simulink model "FlightGear_BUS_aerosurface_trim"  (R2017a)
settings: Solver=VariableStepAuto  StartTime=0.0  StopTime=20  FixedStep=0.1  RelTol=1e-5
model workspace (MAT data in the model file):
  op_trim2 : opcond.OperatingReport (value not decoded)
  op_trim3 : opcond.OperatingReport (value not decoded)
values from neighbouring files (symbols this model uses):
  a0_s2345 = [0;0;0.05;0.05]    [HW5_4_surfaces.m]    (also in TEST_aerosetup.m; surfaces_setup_test.m)
  A_2345 = c_2345.*b_2345    [HW5_4_surfaces.m]    (also in TEST_aerosetup.m; surfaces_setup_test.m)
  Aileron_left = 0    [HW5_4_surfaces.m]    (also in TEST_aerosetup.m; surfaces_setup_test.m)
  Aileron_right = 0    [HW5_4_surfaces.m]    (also in TEST_aerosetup.m; surfaces_setup_test.m)
  c_2345 = [0.075;0.08;0.1;0.1]    [HW5_4_surfaces.m]    (also in TEST_aerosetup.m; surfaces_setup_test.m)
  CD0_s2345 = [0.01;0.01;0.01;0.01]    [HW5_4_surfaces.m]    (also in TEST_aerosetup.m; surfaces_setup_test.m)
  CDa_s2345 = [1;1;1;1]    [HW5_4_surfaces.m]    (also in TEST_aerosetup.m; surfaces_setup_test.m)
  CL0_2345 = [0;0; 0.05; 0.05]    [HW5_4_surfaces.m]    (also in TEST_aerosetup.m; surfaces_setup_test.m)
  CLa = 2*pi*(r./(2+r))    [HW5_4_surfaces.m]    (also in TEST_aerosetup.m; surfaces_setup_test.m)
  CM0_s2345 = [0;0;-0.05;-0.05]    [HW5_4_surfaces.m]    (also in TEST_aerosetup.m; surfaces_setup_test.m)
  CMa_s2345 = [0; 0; 0; 0]    [HW5_4_surfaces.m]    (also in TEST_aerosetup.m; surfaces_setup_test.m)
  e_s2345 = [0.8;0.8;0.9;0.9]    [HW5_4_surfaces.m]    (also in TEST_aerosetup.m; surfaces_setup_test.m)
  elevator = 0    [HW5_4_surfaces.m]    (also in TEST_aerosetup.m; surfaces_setup_test.m)
  Fext_N = -g_EN * m    [HW5_4_surfaces.m]    (also in TEST_aerosetup.m = [10 10 10]; surfaces_setup_test.m)
  g_EN = [0; 0; 9.81]    [HW5_4_surfaces.m]    (also in TEST_aerosetup.m = [0; 0; 9.8]; surfaces_setup_test.m)
  i_s2345 = [0; 0; 0.05; 0.05;]    [HW5_4_surfaces.m]    (also in TEST_aerosetup.m; surfaces_setup_test.m)
  J_cg = ones(3)    [HW5_4_surfaces.m]    (also in TEST_aerosetup.m)
  J_cgp = ones(3)    [surfaces_setup_test.m]
  M_total = sum(MnG(:,1))/1000    [HW5_4_surfaces.m]    (also in TEST_aerosetup.m; surfaces_setup_test.m = sum(MnG1(:,1))/1000)
  Mext_B = [0; 0; 0]    [HW5_4_surfaces.m]    (also in TEST_aerosetup.m = [1; 1; 1]; surfaces_setup_test.m)
  p_E_BE_ini = p_E_BE_ini_deg .* [deg2rad; deg2rad; 1]    [HW5_4_surfaces.m]    (also in TEST_aerosetup.m; surfaces_setup_test.m)
  r = b_2345./c_2345    [HW5_4_surfaces.m]    (also in TEST_aerosetup.m; surfaces_setup_test.m)
  Rearth = 6371000    [HW5_4_surfaces.m]    (also in TEST_aerosetup.m; surfaces_setup_test.m)
  rudder = 0    [HW5_4_surfaces.m]    (also in TEST_aerosetup.m; surfaces_setup_test.m)
  Theta_ini = Theta_ini_deg * deg2rad    [HW5_4_surfaces.m]    (also in TEST_aerosetup.m; surfaces_setup_test.m)
  v_N_AE = [0;0;0]    [HW5_4_surfaces.m]    (also in TEST_aerosetup.m; surfaces_setup_test.m)
  Vbbe_int = [10; 0; 0]    [HW5_4_surfaces.m]    (also in TEST_aerosetup.m; surfaces_setup_test.m = [5; 0; 0])
  w_B_BE_ini = [1e0; 1e-2; 1e-2]    [HW5_4_surfaces.m]    (also in TEST_aerosetup.m; surfaces_setup_test.m)
  xyz_s = [[-0.76 0 0.16];[-0.76 0 -0.09];[-0.23 0.44 0];[-0.23 -0.44 0];]    [HW5_4_surfaces.m]    (also in TEST_aerosetup.m; surfaces_setup_test.m)
undefined symbols (not defined in the file or in its folder): Earth, WGS84
libraries: dspinverses x6, vrlib x4, simulink x4, aerolibfltsims x3, sharedtransform x2, aerolibtransform2 x2, aerolibutil x1, sharedutil x1
(part 1 of 2)
settings Model: Creator=Jiaoran Wang  LastModifiedBy=Jiaoran Wang
settings DataIOCC: ExternalInput=getinputstruct(op_trim3)  InitialState=getstatestruct(op_trim3)  LoadExternalInput=on  LoadInitialState=on

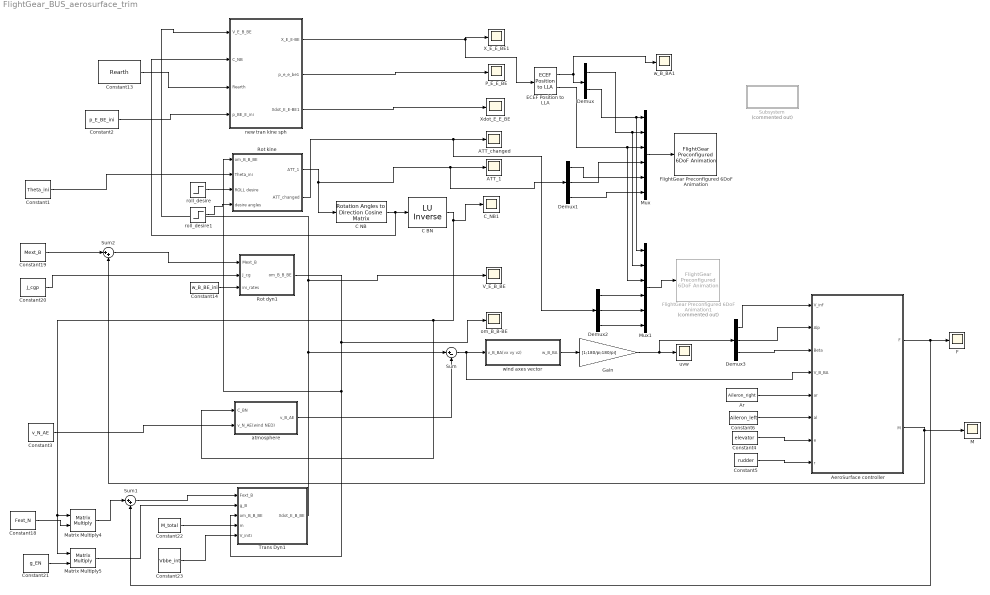
== system FlightGear_BUS_aerosurface_trim ==
  ATT_1 : Scope
  ATT_changed : Scope
  AeroSurface controller : Subsystem
  Ar : Constant  Value=Aileron_right
  C BN : dspinverses/ LU Inverse
      settings: SourceProductName=DSP System Toolbox
  C NB : sharedtransform/Rotation Angles to Direction Cosine Matrix  rotationOrder=ZYX
  C_NB1 : Scope
  Constant1 : Constant  Value=Theta_ini
  Constant13 : Constant  Value=Rearth
  Constant14 : Constant  Value=w_B_BE_ini
  Constant18 : Constant  Value=Fext_N
  Constant19 : Constant  Value=Mext_B
  Constant2 : Constant  Value=p_E_BE_ini  VectorParams1D=off
  Constant20 : Constant  Value=J_cgp
  Constant21 : Constant  Value=g_EN
  Constant22 : Constant  Value=M_total
  Constant23 : Constant  Value=Vbbe_int
  Constant3 : Constant  Value=v_N_AE
  Constant4 : Constant  Value=elevator
  Constant5 : Constant  Value=rudder
  Constant6 : Constant  Value=Aileron_left
  Demux : Demux  Outputs=2
  Demux1 : Demux  Outputs=3
  Demux2 : Demux  Outputs=3
  Demux3 : Demux  Outputs=3
  ECEF Position to LLA : aerolibtransform2/ECEF Position to LLA  units=Metric (MKS)  ptype=Earth (WGS84)  F=1/298.257223563  R=6378137
      settings: SourceProductName=Aerospace Blockset  SourceProductBaseCode=AE
  F : Scope
  FlightGear Preconfigured 6DoF Animation : aerolibfltsims/FlightGear Preconfigured 6DoF Animation  xFlightGearVersion=v3.0  DestinationIpAddress=127.0.0.1  DestinationPort=5502  SampleTime=1/50
      settings: SourceProductName=Aerospace Blockset
  FlightGear Preconfigured 6DoF Animation1 : aerolibfltsims/FlightGear Preconfigured 6DoF Animation  Commented=on  xFlightGearVersion=v3.0  DestinationIpAddress=127.0.0.1  DestinationPort=5502  SampleTime=1/50
      settings: SourceProductName=Aerospace Blockset
  Gain : Gain  Gain=[1;180/pi;180/pi]
  M : Scope
  Matrix Multiply4 : Product  Multiplication=Matrix(*)
  Matrix Multiply5 : Product  Multiplication=Matrix(*)
  Mux : Mux  Inputs=6
  Mux1 : Mux  Inputs=6
  P_E_E_BE : Scope
  Rot dyn1 : Subsystem
  Rot kine : Subsystem
  Subsystem : Subsystem  Commented=on
  Sum : Sum  Inputs=|+-
  Sum1 : Sum  Inputs=|++
  Sum2 : Sum  Inputs=|++
  Trans Dyn1 : Subsystem
  V_E_B_BE : Scope
  "X_E_E_BE1 " : Scope
  Xdot_E_E_BE : Scope
  atmosphere : Subsystem
  new tran kine sph : Subsystem
  om_B_B-BE : Scope
  roll_desire : Step  Time=0  After=0  SampleTime=0
  roll_desire1 : Step  Time=0  After=0  SampleTime=0
  uvw : Scope
  w_B_BA1 : Scope
  wind axes vector : Subsystem
  wires:
  ECEF Position to LLA/1 -> Demux/1, w_B_BA1/1
  Constant2/1 -> new tran kine sph/4(p_BE_E_ini)
  Constant13/1 -> new tran kine sph/3(Rearth)
  C BN/1 -> C_NB1/1, atmosphere/1(C_BN), Matrix Multiply5/1, Matrix Multiply4/1
  Matrix Multiply5/1 -> Trans Dyn1/2(g_B)
  Demux/1 -> Mux1/2, Mux/2
  new tran kine sph/2(p_e_e_be1) -> P_E_E_BE/1
  Constant23/1 -> Trans Dyn1/5(V_initi)
  ECEF Position to LLA/2 -> Mux1/3, Mux/3
  Constant18/1 -> Matrix Multiply4/2
  wind axes vector/1(w_B_BA) -> Gain/1
  atmosphere/1(v_B_AE) -> Sum/2
  Demux/2 -> Mux1/1, Mux/1
  Constant3/1 -> atmosphere/2(v_N_AE(wind NED))
  new tran kine sph/1(X_E_E-BE) -> "X_E_E_BE1 "/1, ECEF Position to LLA/1
  new tran kine sph/3(Xdot_E_E-BE1) -> Xdot_E_E_BE/1
  Rot dyn1/1(om_B_B_BE) -> Trans Dyn1/3(om_B_B_BE), Rot kine/1(om_B_B_BE), om_B_B-BE/1
  Constant14/1 -> Rot dyn1/3(ini_rates)
  Constant1/1 -> Rot kine/2(Theta_ini)
  Trans Dyn1/1(Xdot_E_B_BE) -> new tran kine sph/1(V_E_B_BE), V_E_B_BE/1, Sum/1
  Constant22/1 -> Trans Dyn1/4(m)
  Constant21/1 -> Matrix Multiply5/2
  C NB/1 -> new tran kine sph/2(C_NB), C BN/1
  Rot kine/1(ATT_1) -> Demux1/1, ATT_1/1, C NB/1
  Constant20/1 -> Rot dyn1/2(J_cg)
  Mux/1 -> FlightGear Preconfigured 6DoF Animation/1
  Demux1/3 -> Mux/6
  Rot kine/2(ATT_changed) -> Demux2/1, ATT_changed/1
  roll_desire/1 -> Rot kine/3(ROLL desire)
  roll_desire1/1 -> Rot kine/4(" desire angles")
  Mux1/1 -> FlightGear Preconfigured 6DoF Animation1/1
  Demux2/3 -> Mux1/6
  Demux2/2 -> Mux1/5
  Demux2/1 -> Mux1/4
  Demux1/2 -> Mux/4
  Demux1/1 -> Mux/5
  Gain/1 -> Demux3/1, uvw/1
  Demux3/1 -> AeroSurface controller/1(V_inf)
  Demux3/2 -> AeroSurface controller/2(Alp)
  Demux3/3 -> AeroSurface controller/3(Beta)
  Sum/1 -> AeroSurface controller/4(V_B_BA), wind axes vector/1(v_B_BA(vx vy vz))
  Constant4/1 -> AeroSurface controller/7(e)
  Constant5/1 -> AeroSurface controller/8(r)
  Ar/1 -> AeroSurface controller/5(ar)
  Constant6/1 -> AeroSurface controller/6(al)
  AeroSurface controller/2(M) -> M/1, Sum2/2
  Matrix Multiply4/1 -> Sum1/1
  Sum1/1 -> Trans Dyn1/1(Fext_B)
  AeroSurface controller/1(F) -> F/1, Sum1/2
  Constant19/1 -> Sum2/1
  Sum2/1 -> Rot dyn1/1(Mext_B)

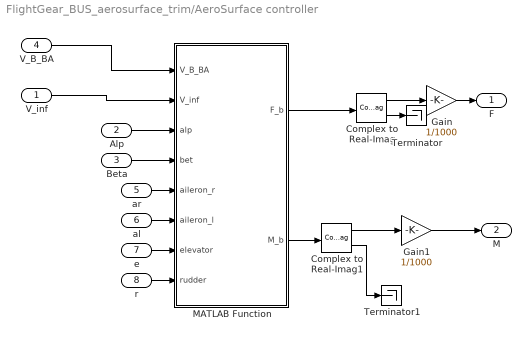
== system FlightGear_BUS_aerosurface_trim/AeroSurface controller ==
  V_inf : Inport
  Alp : Inport  Port=2
  Beta : Inport  Port=3
  V_B_BA : Inport  Port=4
  ar : Inport  Port=5
  al : Inport  Port=6
  e : Inport  Port=7
  r : Inport  Port=8
  Complex to Real-Imag : ComplexToRealImag
  Complex to Real-Imag1 : ComplexToRealImag
  Gain : Gain  Gain=1/1000
  Gain1 : Gain  Gain=1/1000
  MATLAB Function : MATLAB Function  TreatAsAtomicUnit=on
  Terminator : Terminator
  Terminator1 : Terminator
  F : Outport
  M : Outport  Port=2
  wires:
  V_inf/1 -> MATLAB Function/2(V_inf)
  V_B_BA/1 -> MATLAB Function/1(V_B_BA)
  ar/1 -> MATLAB Function/5(aileron_r)
  al/1 -> MATLAB Function/6(aileron_l)
  e/1 -> MATLAB Function/7(elevator)
  r/1 -> MATLAB Function/8(rudder)
  Alp/1 -> MATLAB Function/3(alp)
  Beta/1 -> MATLAB Function/4(bet)
  MATLAB Function/1(F_b) -> Complex to Real-Imag/1
  Complex to Real-Imag/1 -> Gain/1
  Complex to Real-Imag/2 -> Terminator/1
  MATLAB Function/2(M_b) -> Complex to Real-Imag1/1
  Complex to Real-Imag1/2 -> Terminator1/1
  Complex to Real-Imag1/1 -> Gain1/1
  Gain/1 -> F/1
  Gain1/1 -> M/1

== system FlightGear_BUS_aerosurface_trim/Rot dyn1 ==
  Mext_B : Inport
  J_cg : Inport  Port=2
  ini_rates : Inport  Port=3
  " LU Inverse" : dspinverses/ LU Inverse
      settings: SourceProductName=DSP System Toolbox
  Add : Sum  Inputs=+-
  Cross Product : vrlib/Utilities/Cross Product
      settings: SourceProductBaseCode=VR
  Integrator : Integrator  InitialConditionSource=external
  Matrix Multiply : Product  Multiplication=Matrix(*)
  Matrix Multiply1 : Product  Multiplication=Matrix(*)
  om_B_B_BE : Outport
  wires:
  J_cg/1 -> " LU Inverse"/1, Matrix Multiply/1
  Matrix Multiply/1 -> Cross Product/2
  " LU Inverse"/1 -> Matrix Multiply1/1
  Add/1 -> Matrix Multiply1/2
  Cross Product/1 -> Add/2
  Matrix Multiply1/1 -> Integrator/1
  ini_rates/1 -> Integrator/2
  Integrator/1 -> Cross Product/1, Matrix Multiply/2, om_B_B_BE/1
  Mext_B/1 -> Add/1

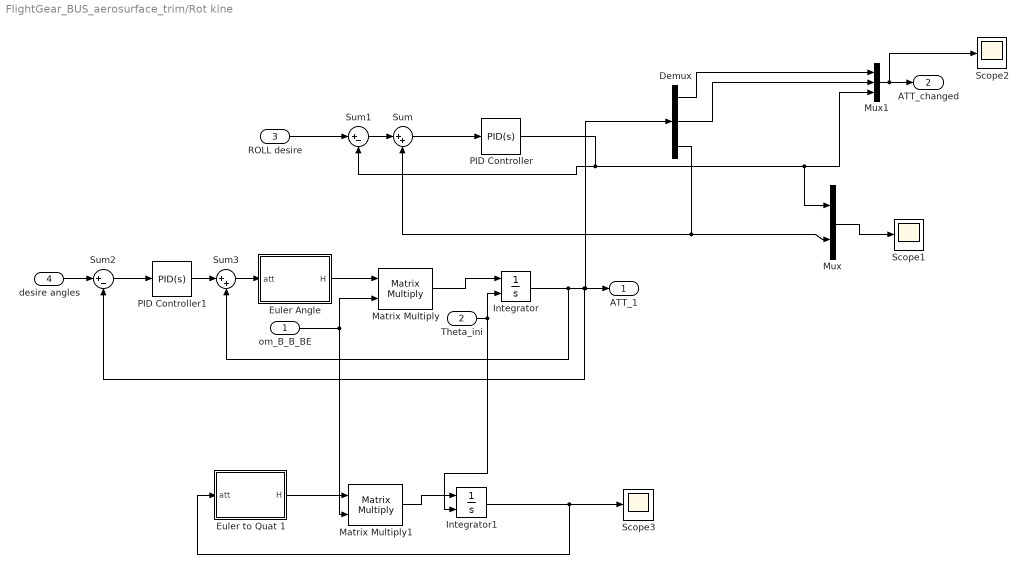
== system FlightGear_BUS_aerosurface_trim/Rot kine ==
  om_B_B_BE : Inport
  Theta_ini : Inport  Port=2
  ROLL desire : Inport  Port=3
  " desire angles" : Inport  Port=4
  Demux : Demux  Outputs=3
  "Euler Angle " : MATLAB Function  TreatAsAtomicUnit=on
  Euler to Quat 1 : MATLAB Function  TreatAsAtomicUnit=on
  Integrator : Integrator  InitialConditionSource=external
  Integrator1 : Integrator  InitialConditionSource=external
  Matrix Multiply : Product  Multiplication=Matrix(*)
  Matrix Multiply1 : Product  Multiplication=Matrix(*)
  Mux : Mux  Inputs=2
  Mux1 : Mux  Inputs=3
  PID Controller : simulink/Continuous/PID Controller  Controller=PID  TimeDomain=Continuous-time  SampleTime=-1  IntegratorMethod=Forward Euler  FilterMethod=Forward Euler  Form=Parallel  UseFilter=on  ControllerParametersSource=internal  P=0  I=10  D=0  N=100  InitialConditionSource=internal  InitialConditionForIntegrator=0  InitialConditionForFilter=0  ExternalReset=none  LimitOutput=off  UpperSaturationLimit=inf  LowerSaturationLimit=-inf  LinearizeAsGain=on  AntiWindupMode=none  Kb=1  TrackingMode=off  Kt=1  PParamMin=[]  PParamMax=[]  IParamMin=[]  IParamMax=[]  DParamMin=[]  DParamMax=[]  NParamMin=[]  NParamMax=[]  KbParamMin=[]  KbParamMax=[]  KtParamMin=[]  KtParamMax=[]  POutMin=[]  POutMax=[]  IOutMin=[]  IOutMax=[]  DOutMin=[]  DOutMax=[]  NOutMin=[]  NOutMax=[]  KbOutMin=[]  KbOutMax=[]  KtOutMin=[]  KtOutMax=[]  IntegratorOutMin=[]  IntegratorOutMax=[]  FilterOutMin=[]  FilterOutMax=[]  SumOutMin=[]  SumOutMax=[]  SumI1OutMin=[]  SumI1OutMax=[]  SumI2OutMin=[]  SumI2OutMax=[]  SumI3OutMin=[]  SumI3OutMax=[]  SumDOutMin=[]  SumDOutMax=[]  SaturationOutMin=[]  SaturationOutMax=[]  IntegratorContinuousStateAttributes=''  IntegratorStateMustResolveToSignalObject=off  IntegratorRTWStateStorageClass=Auto  FilterContinuousStateAttributes=''  FilterStateMustResolveToSignalObject=off  FilterRTWStateStorageClass=Auto  DifferentiatorICPrevScaledInput=0  DifferentiatorOutMin=[]  DifferentiatorOutMax=[]  InitialConditionSetting=State (most efficient)
  PID Controller1 : simulink/Continuous/PID Controller  Controller=PID  TimeDomain=Continuous-time  SampleTime=-1  IntegratorMethod=Forward Euler  FilterMethod=Forward Euler  Form=Parallel  UseFilter=on  ControllerParametersSource=internal  P=0  I=10  D=0  N=100  InitialConditionSource=internal  InitialConditionForIntegrator=0  InitialConditionForFilter=0  ExternalReset=none  LimitOutput=off  UpperSaturationLimit=inf  LowerSaturationLimit=-inf  LinearizeAsGain=on  AntiWindupMode=none  Kb=1  TrackingMode=off  Kt=1  PParamMin=[]  PParamMax=[]  IParamMin=[]  IParamMax=[]  DParamMin=[]  DParamMax=[]  NParamMin=[]  NParamMax=[]  KbParamMin=[]  KbParamMax=[]  KtParamMin=[]  KtParamMax=[]  POutMin=[]  POutMax=[]  IOutMin=[]  IOutMax=[]  DOutMin=[]  DOutMax=[]  NOutMin=[]  NOutMax=[]  KbOutMin=[]  KbOutMax=[]  KtOutMin=[]  KtOutMax=[]  IntegratorOutMin=[]  IntegratorOutMax=[]  FilterOutMin=[]  FilterOutMax=[]  SumOutMin=[]  SumOutMax=[]  SumI1OutMin=[]  SumI1OutMax=[]  SumI2OutMin=[]  SumI2OutMax=[]  SumI3OutMin=[]  SumI3OutMax=[]  SumDOutMin=[]  SumDOutMax=[]  SaturationOutMin=[]  SaturationOutMax=[]  IntegratorContinuousStateAttributes=''  IntegratorStateMustResolveToSignalObject=off  IntegratorRTWStateStorageClass=Auto  FilterContinuousStateAttributes=''  FilterStateMustResolveToSignalObject=off  FilterRTWStateStorageClass=Auto  DifferentiatorICPrevScaledInput=0  DifferentiatorOutMin=[]  DifferentiatorOutMax=[]  InitialConditionSetting=State (most efficient)
  Scope1 : Scope
  Scope2 : Scope
  Scope3 : Scope
  Sum : Sum  Inputs=|++
  Sum1 : Sum  Inputs=|+-
  Sum2 : Sum  Inputs=|+-
  Sum3 : Sum  Inputs=|++
  ATT_1 : Outport
  ATT_changed : Outport  Port=2
  wires:
  om_B_B_BE/1 -> Matrix Multiply1/2, Matrix Multiply/2
  Integrator/1 -> ATT_1/1, Demux/1, Sum2/2, Sum3/2
  "Euler Angle "/1(H) -> Matrix Multiply/1
  Theta_ini/1 -> Integrator/2, Integrator1/2
  Matrix Multiply/1 -> Integrator/1
  Demux/3 -> Sum/2, Mux/2
  Demux/1 -> Mux1/1
  PID Controller/1 -> Sum1/2, Mux/1, Mux1/3
  Mux/1 -> Scope1/1
  Demux/2 -> Mux1/2
  Mux1/1 -> Scope2/1, ATT_changed/1
  ROLL desire/1 -> Sum1/1
  Sum1/1 -> Sum/1
  Sum/1 -> PID Controller/1
  Sum2/1 -> PID Controller1/1
  " desire angles"/1 -> Sum2/1
  PID Controller1/1 -> Sum3/1
  Sum3/1 -> "Euler Angle "/1(att)
  Integrator1/1 -> Euler to Quat 1/1(att), Scope3/1
  Matrix Multiply1/1 -> Integrator1/1
  Euler to Quat 1/1(H) -> Matrix Multiply1/1

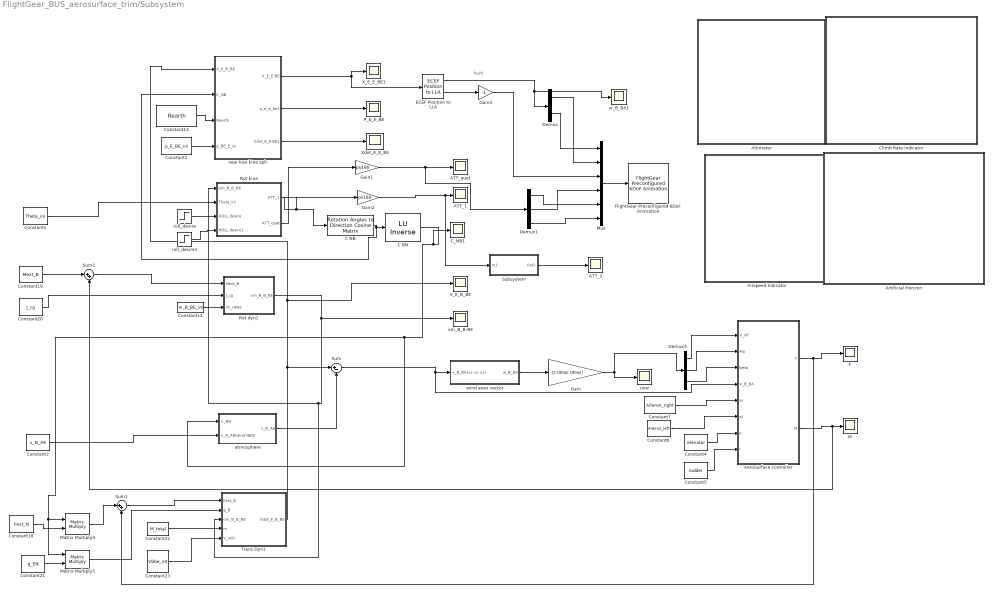
== system FlightGear_BUS_aerosurface_trim/Subsystem ==
  note: hurh
  ATT_1 : Scope
  ATT_2 : Scope
  ATT_quat : Scope
  AeroSurface controller : Subsystem
  Airspeed Indicator : Subsystem  DialogController=aeroblksHMICreateDDGDialog  IsWebBlock=on  mask(MWDashboardBlock){webBlockId=e5e3171d-ff29-4451-bf74-d38876eec561, webBlockType=airspeedindicator, ShowInLibBrowser=on, ShowInitialText=on, HMISrcModelName=[]}
      mask prompts: webBlockId "WebBlock Id"; webBlockType "WebBlock Type"; HMISrcModelName "Source Model"
      mask help: aeroblksHMI:aeroblkhmi:AirspeedIndicatorDialogDesc
      mask Help: eval('asbhmihelp(''airspeedindicator'')');
      mask Display:
      | if strcmp(get_param(bdroot(gcb),'BlockDiagramType'), 'library')
      |  image([(matlabroot) '/toolbox/aeroblks/aeroblks/hmi/icons/AirspeedIndicatorIcon.svg'])
      | end
  Altimeter : Subsystem  DialogController=aeroblksHMICreateDDGDialog  IsWebBlock=on  mask(MWDashboardBlock){webBlockId=36990637-e96a-433a-956a-f44ed4ed9d1e, webBlockType=altimeter, ShowInLibBrowser=on, ShowInitialText=on, HMISrcModelName=[]}
      mask prompts: webBlockId "WebBlock Id"; webBlockType "WebBlock Type"; HMISrcModelName "Source Model"
      mask help: aeroblksHMI:aeroblkhmi:AltimeterDialogDesc
      mask Help: eval('asbhmihelp(''altimeter'')');
      mask Display:
      | if strcmp(get_param(bdroot(gcb),'BlockDiagramType'), 'library')
      |  image([(matlabroot) '/toolbox/aeroblks/aeroblks/hmi/icons/AltimeterIcon.svg'])
      | end
  Artificial Horizon : Subsystem  DialogController=aeroblksHMICreateDDGDialog  IsWebBlock=on  mask(MWDashboardBlock){webBlockId=4cd5d09c-38f7-433d-892c-50154f5485b8, webBlockType=artificialhorizon, ShowInLibBrowser=on, ShowInitialText=on, HMISrcModelName=[]}
      mask prompts: webBlockId "WebBlock Id"; webBlockType "WebBlock Type"; HMISrcModelName "Source Model"
      mask help: aeroblksHMI:aeroblkhmi:ArtificialHorizonDialogDesc
      mask Help: eval('asbhmihelp(''artificialhorizon'')');
      mask Display:
      | if strcmp(get_param(bdroot(gcb),'BlockDiagramType'), 'library')
      |  image([(matlabroot) '/toolbox/aeroblks/aeroblks/hmi/icons/ArtificialHorizonIcon.svg'])
      | end
  C BN : dspinverses/ LU Inverse
      settings: SourceProductName=DSP System Toolbox
  C NB : sharedtransform/Rotation Angles to Direction Cosine Matrix  rotationOrder=ZYX
  C_NB1 : Scope
  Climb Rate Indicator : Subsystem  DialogController=aeroblksHMICreateDDGDialog  IsWebBlock=on  mask(MWDashboardBlock){webBlockId=79e6d40e-4c73-4bf3-981b-23b4e158f69b, webBlockType=climbindicator, ShowInLibBrowser=on, ShowInitialText=on, HMISrcModelName=[]}
      mask prompts: webBlockId "WebBlock Id"; webBlockType "WebBlock Type"; HMISrcModelName "Source Model"
      mask help: aeroblksHMI:aeroblkhmi:ClimbIndicatorDialogDesc
      mask Help: eval('asbhmihelp(''climbindicator'')');
      mask Display:
      | if strcmp(get_param(bdroot(gcb),'BlockDiagramType'), 'library')
      |  image([(matlabroot) '/toolbox/aeroblks/aeroblks/hmi/icons/ClimbIndicatorIcon.svg'])
      | end
  Constant1 : Constant  Value=Theta_ini
  Constant13 : Constant  Value=Rearth
  Constant14 : Constant  Value=w_B_BE_ini
  Constant18 : Constant  Value=Fext_N
  Constant19 : Constant  Value=Mext_B
  Constant2 : Constant  Value=p_E_BE_ini  VectorParams1D=off
  Constant20 : Constant  Value=J_cg
  Constant21 : Constant  Value=g_EN
  Constant22 : Constant  Value=M_total
  Constant23 : Constant  Value=Vbbe_int
  Constant3 : Constant  Value=v_N_AE
  Constant4 : Constant  Value=elevator
  Constant5 : Constant  Value=rudder
  Constant6 : Constant  Value=Aileron_left
  Constant7 : Constant  Value=Aileron_right
  Demux : Demux  Outputs=2
  Demux1 : Demux  Outputs=3
  Demux3 : Demux  Outputs=3
  ECEF Position to LLA : aerolibtransform2/ECEF Position to LLA  units=Metric (MKS)  ptype=Earth (WGS84)  F=1/298.257223563  R=6378137
      settings: SourceProductName=Aerospace Blockset  SourceProductBaseCode=AE
  F : Scope
  FlightGear Preconfigured 6DoF Animation : aerolibfltsims/FlightGear Preconfigured 6DoF Animation  xFlightGearVersion=v3.0  DestinationIpAddress=127.0.0.1  DestinationPort=5502  SampleTime=1/50
      settings: SourceProductName=Aerospace Blockset
  Gain : Gain  Gain=[1;180/pi;180/pi]
  Gain1 : Gain  Gain=pi/180
  Gain2 : Gain  Gain=pi/180
  Gain3 : Gain  Gain=-1
  M : Scope
  Matrix Multiply4 : Product  Multiplication=Matrix(*)
  Matrix Multiply5 : Product  Multiplication=Matrix(*)
  Mux : Mux  Inputs=6
  P_E_E_BE : Scope
  Rot dyn1 : Subsystem
  Rot kine : Subsystem
  Subsystem : Subsystem
  Sum : Sum  Inputs=|+-
  Sum1 : Sum  Inputs=|++
  Sum2 : Sum  Inputs=|++
  Trans Dyn1 : Subsystem
  V_E_B_BE : Scope
  "X_E_E_BE1 " : Scope
  Xdot_E_E_BE : Scope
  atmosphere : Subsystem
  new tran kine sph : Subsystem
  om_B_B-BE : Scope
  roll_desire : Step  Time=0  After=0  SampleTime=0
  roll_desire1 : Step  Time=0  After=0  SampleTime=0
  uvw : Scope
  w_B_BA1 : Scope
  wind axes vector : Subsystem
  wires:
  Subsystem/1(Out1) -> ATT_2/1
  Demux3/3 -> AeroSurface controller/3(Beta)
  Rot kine/1(ATT_1) -> C NB/1, Gain2/1
  Gain1/1 -> Demux1/1, ATT_quat/1
  C BN/1 -> atmosphere/1(C_BN), Matrix Multiply5/1, Matrix Multiply4/1, C_NB1/1
  Constant19/1 -> Sum2/1
  Gain3/1 -> Mux/3
  Constant7/1 -> AeroSurface controller/5(ar)
  Gain2/1 -> Subsystem/1(In1), ATT_1/1
  Mux/1 -> FlightGear Preconfigured 6DoF Animation/1
  Rot kine/2(ATT_quat) -> Gain1/1
  Sum2/1 -> Rot dyn1/1(Mext_B)
  Sum1/1 -> Trans Dyn1/1(Fext_B)
  wind axes vector/1(w_B_BA) -> Gain/1
  AeroSurface controller/1(F) -> Sum1/2, F/1
  Rot dyn1/1(om_B_B_BE) -> Trans Dyn1/3(om_B_B_BE), Rot kine/1(om_B_B_BE), om_B_B-BE/1
  Demux1/3 -> Mux/6
  Demux3/2 -> AeroSurface controller/2(Alp)
  Constant21/1 -> Matrix Multiply5/2
  Constant5/1 -> AeroSurface controller/8(r)
  Constant22/1 -> Trans Dyn1/4(m)
  Constant2/1 -> new tran kine sph/4(p_BE_E_ini)
  Demux/1 -> Mux/2
  Sum/1 -> AeroSurface controller/4(V_B_BA), wind axes vector/1(v_B_BA(vx vy vz))
  Demux1/1 -> Mux/5
  Constant4/1 -> AeroSurface controller/7(e)
  Constant1/1 -> Rot kine/2(Theta_ini)
  Constant23/1 -> Trans Dyn1/5(V_initi)
  Gain/1 -> Demux3/1, uvw/1
  C NB/1 -> new tran kine sph/2(C_NB), C BN/1
  atmosphere/1(v_B_AE) -> Sum/2
  Constant18/1 -> Matrix Multiply4/2
  ECEF Position to LLA/2 -> Gain3/1
  Demux/2 -> Mux/1
  Demux3/1 -> AeroSurface controller/1(V_inf)
  Constant13/1 -> new tran kine sph/3(Rearth)
  new tran kine sph/1(X_E_E-BE) -> ECEF Position to LLA/1, "X_E_E_BE1 "/1
  new tran kine sph/2(p_e_e_be1) -> P_E_E_BE/1
  Constant3/1 -> atmosphere/2(v_N_AE(wind NED))
  Constant14/1 -> Rot dyn1/3(ini_rates)
  Demux1/2 -> Mux/4
  new tran kine sph/3(Xdot_E_E-BE1) -> Xdot_E_E_BE/1
  roll_desire1/1 -> Rot kine/4(ROLL desire1)
  AeroSurface controller/2(M) -> Sum2/2, M/1
  Constant6/1 -> AeroSurface controller/6(al)
  Matrix Multiply4/1 -> Sum1/1
  roll_desire/1 -> Rot kine/3(ROLL desire)
  Trans Dyn1/1(Xdot_E_B_BE) -> new tran kine sph/1(V_E_B_BE), V_E_B_BE/1, Sum/1
  Matrix Multiply5/1 -> Trans Dyn1/2(g_B)
  ECEF Position to LLA/1 -> Demux/1, w_B_BA1/1
  Constant20/1 -> Rot dyn1/2(J_cg)

== system FlightGear_BUS_aerosurface_trim/Trans Dyn1 ==
  Fext_B : Inport
  g_B : Inport  Port=2
  om_B_B_BE : Inport  Port=3
  m : Inport  Port=4
  V_initi : Inport  Port=5
  Add : Sum  Inputs=++-
  Cross Product : vrlib/Utilities/Cross Product
      settings: SourceProductBaseCode=VR
  Divide : Product  Inputs=*/
  Integrator : Integrator  InitialConditionSource=external
  Xdot_E_B_BE : Outport
  wires:
  Fext_B/1 -> Divide/1
  m/1 -> Divide/2
  Divide/1 -> Add/1
  g_B/1 -> Add/2
  om_B_B_BE/1 -> Cross Product/1
  Cross Product/1 -> Add/3
  Add/1 -> Integrator/1
  V_initi/1 -> Integrator/2
  Integrator/1 -> Cross Product/2, Xdot_E_B_BE/1

== system FlightGear_BUS_aerosurface_trim/atmosphere ==
  C_BN : Inport
  v_N_AE(wind NED) : Inport  Port=2
  Matrix Multiply : Product  Multiplication=Matrix(*)
  v_B_AE : Outport
  wires:
  v_N_AE(wind NED)/1 -> Matrix Multiply/2
  C_BN/1 -> Matrix Multiply/1
  Matrix Multiply/1 -> v_B_AE/1

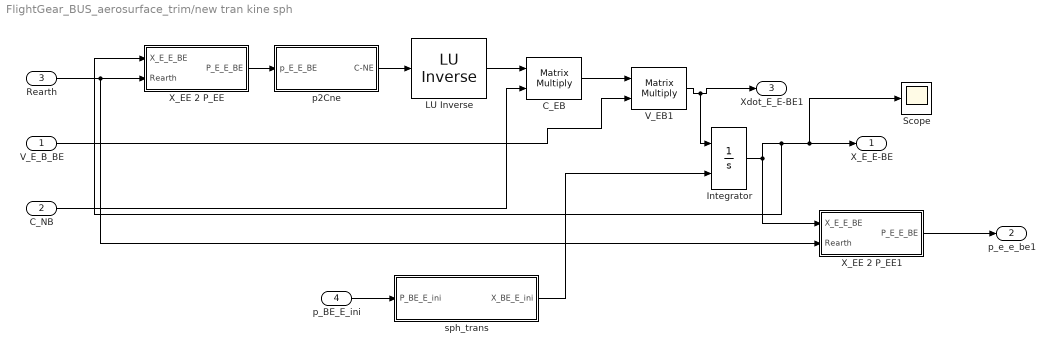
== system FlightGear_BUS_aerosurface_trim/new tran kine sph ==
  V_E_B_BE : Inport
  C_NB : Inport  Port=2
  Rearth : Inport  Port=3
  p_BE_E_ini : Inport  Port=4
  " LU Inverse" : dspinverses/ LU Inverse
      settings: SourceProductName=DSP System Toolbox
  C_EB : Product  Multiplication=Matrix(*)
  Integrator : Integrator  InitialConditionSource=external
  Scope : Scope
  V_EB1 : Product  Multiplication=Matrix(*)
  X_EE 2 P_EE : Subsystem
  X_EE 2 P_EE1 : Subsystem
  p2Cne : Subsystem
  sph_trans : MATLAB Function  TreatAsAtomicUnit=on
  X_E_E-BE : Outport
  p_e_e_be1 : Outport  Port=2
  Xdot_E_E-BE1 : Outport  Port=3
  wires:
  " LU Inverse"/1 -> C_EB/1
  Integrator/1 -> Scope/1, X_E_E-BE/1, X_EE 2 P_EE/1(X_E_E_BE), X_EE 2 P_EE1/1(X_E_E_BE)
  X_EE 2 P_EE1/1(P_E_E_BE) -> p_e_e_be1/1
  Rearth/1 -> X_EE 2 P_EE1/2(Rearth), X_EE 2 P_EE/2(Rearth)
  V_EB1/1 -> Xdot_E_E-BE1/1, Integrator/1
  C_EB/1 -> V_EB1/1
  p2Cne/1(C-NE) -> " LU Inverse"/1
  X_EE 2 P_EE/1(P_E_E_BE) -> p2Cne/1(p_E_E_BE)
  C_NB/1 -> C_EB/2
  V_E_B_BE/1 -> V_EB1/2
  p_BE_E_ini/1 -> sph_trans/1(P_BE_E_ini)
  sph_trans/1(X_BE_E_ini) -> Integrator/2

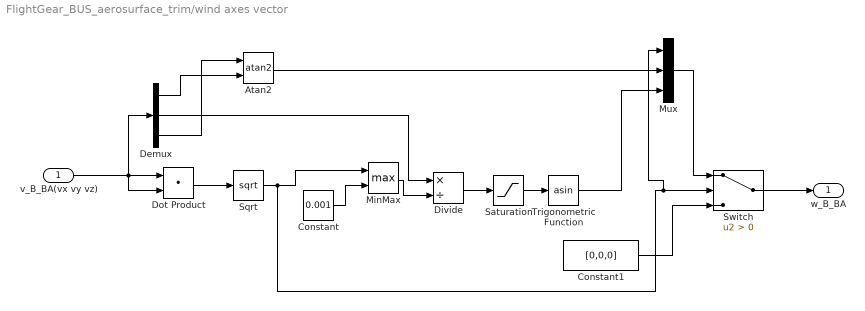
== system FlightGear_BUS_aerosurface_trim/wind axes vector ==
  v_B_BA(vx vy vz) : Inport
  Atan2 : Trigonometry  Operator=atan2
  Constant : Constant  Value=0.001
  Constant1 : Constant  Value=[0,0,0]
  Demux : Demux  Outputs=3
  Divide : Product  Inputs=*/
  Dot Product : DotProduct  InputSameDT=on  OutDataTypeStr=Inherit: Inherit via internal rule
  MinMax : MinMax  Function=max  Inputs=2
  Mux : Mux  Inputs=3
  Saturation : Saturate
  Sqrt : Sqrt  SaturateOnIntegerOverflow=on
  Switch : Switch  Criteria=u2 > Threshold
  Trigonometric Function : Trigonometry  Operator=asin  ApproximationMethod=CORDIC
  w_B_BA : Outport
  wires:
  v_B_BA(vx vy vz)/1 -> Demux/1, Dot Product/2, Dot Product/1
  Dot Product/1 -> Sqrt/1
  Sqrt/1 -> Mux/1, Switch/2, MinMax/1
  Constant/1 -> MinMax/2
  MinMax/1 -> Divide/2
  Demux/2 -> Divide/1
  Demux/3 -> Atan2/1
  Demux/1 -> Atan2/2
  Atan2/1 -> Mux/2
  Divide/1 -> Saturation/1
  Saturation/1 -> Trigonometric Function/1
  Trigonometric Function/1 -> Mux/3
  Constant1/1 -> Switch/3
  Mux/1 -> Switch/1
  Switch/1 -> w_B_BA/1

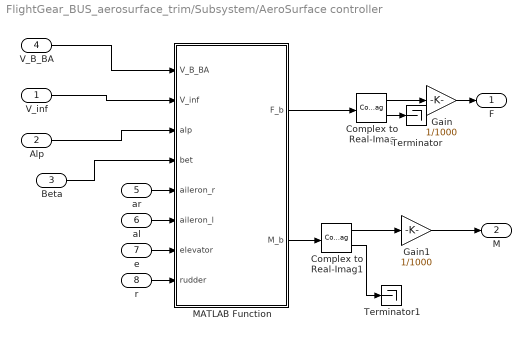
== system FlightGear_BUS_aerosurface_trim/Subsystem/AeroSurface controller ==
  V_inf : Inport
  Alp : Inport  Port=2
  Beta : Inport  Port=3
  V_B_BA : Inport  Port=4
  ar : Inport  Port=5
  al : Inport  Port=6
  e : Inport  Port=7
  r : Inport  Port=8
  Complex to Real-Imag : ComplexToRealImag
  Complex to Real-Imag1 : ComplexToRealImag
  Gain : Gain  Gain=1/1000
  Gain1 : Gain  Gain=1/1000
  MATLAB Function : MATLAB Function  TreatAsAtomicUnit=on
  Terminator : Terminator
  Terminator1 : Terminator
  F : Outport
  M : Outport  Port=2
  wires:
  V_inf/1 -> MATLAB Function/2(V_inf)
  V_B_BA/1 -> MATLAB Function/1(V_B_BA)
  ar/1 -> MATLAB Function/5(aileron_r)
  al/1 -> MATLAB Function/6(aileron_l)
  e/1 -> MATLAB Function/7(elevator)
  r/1 -> MATLAB Function/8(rudder)
  Alp/1 -> MATLAB Function/3(alp)
  Beta/1 -> MATLAB Function/4(bet)
  MATLAB Function/1(F_b) -> Complex to Real-Imag/1
  Complex to Real-Imag/1 -> Gain/1
  Complex to Real-Imag/2 -> Terminator/1
  MATLAB Function/2(M_b) -> Complex to Real-Imag1/1
  Complex to Real-Imag1/2 -> Terminator1/1
  Complex to Real-Imag1/1 -> Gain1/1
  Gain/1 -> F/1
  Gain1/1 -> M/1

== system FlightGear_BUS_aerosurface_trim/Subsystem/Airspeed Indicator ==

== system FlightGear_BUS_aerosurface_trim/Subsystem/Altimeter ==

== system FlightGear_BUS_aerosurface_trim/Subsystem/Artificial Horizon ==

== system FlightGear_BUS_aerosurface_trim/Subsystem/Climb Rate Indicator ==

== system FlightGear_BUS_aerosurface_trim/Subsystem/Rot dyn1 ==
  Mext_B : Inport
  J_cg : Inport  Port=2
  ini_rates : Inport  Port=3
  " LU Inverse" : dspinverses/ LU Inverse
      settings: SourceProductName=DSP System Toolbox
  Add : Sum  Inputs=+-
  Cross Product : vrlib/Utilities/Cross Product
      settings: SourceProductBaseCode=VR
  Integrator : Integrator  InitialConditionSource=external
  Matrix Multiply : Product  Multiplication=Matrix(*)
  Matrix Multiply1 : Product  Multiplication=Matrix(*)
  om_B_B_BE : Outport
  wires:
  J_cg/1 -> " LU Inverse"/1, Matrix Multiply/1
  Matrix Multiply/1 -> Cross Product/2
  " LU Inverse"/1 -> Matrix Multiply1/1
  Add/1 -> Matrix Multiply1/2
  Cross Product/1 -> Add/2
  Matrix Multiply1/1 -> Integrator/1
  ini_rates/1 -> Integrator/2
  Integrator/1 -> Cross Product/1, Matrix Multiply/2, om_B_B_BE/1
  Mext_B/1 -> Add/1

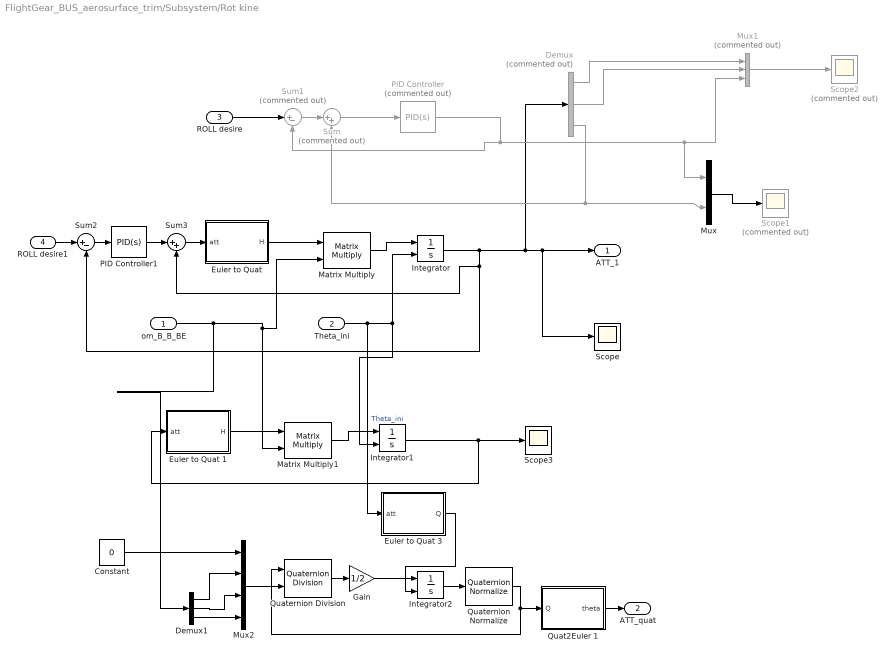
== system FlightGear_BUS_aerosurface_trim/Subsystem/Rot kine ==
  om_B_B_BE : Inport
  Theta_ini : Inport  Port=2
  ROLL desire : Inport  Port=3
  ROLL desire1 : Inport  Port=4
  Constant : Constant  Value=0
  Demux : Demux  Commented=on  Outputs=3
  Demux1 : Demux  Outputs=3
  "Euler to Quat " : MATLAB Function  TreatAsAtomicUnit=on
  Euler to Quat 1 : MATLAB Function  TreatAsAtomicUnit=on
  Euler to Quat 3 : MATLAB Function  TreatAsAtomicUnit=on
  Gain : Gain  Gain=1/2
  Integrator : Integrator  InitialConditionSource=external
  Integrator1 : Integrator  InitialConditionSource=external
  Integrator2 : Integrator  InitialConditionSource=external
  Matrix Multiply : Product  Multiplication=Matrix(*)
  Matrix Multiply1 : Product  Multiplication=Matrix(*)
  Mux : Mux  Inputs=2
  Mux1 : Mux  Commented=on  Inputs=3
  Mux2 : Mux  Inputs=4'
  PID Controller : simulink/Continuous/PID Controller  Commented=on  Controller=PID  TimeDomain=Continuous-time  SampleTime=-1  IntegratorMethod=Forward Euler  FilterMethod=Forward Euler  Form=Parallel  UseFilter=on  ControllerParametersSource=internal  P=0  I=10  D=0  N=100  InitialConditionSource=internal  InitialConditionForIntegrator=0  InitialConditionForFilter=0  ExternalReset=none  LimitOutput=off  UpperSaturationLimit=inf  LowerSaturationLimit=-inf  LinearizeAsGain=on  AntiWindupMode=none  Kb=1  TrackingMode=off  Kt=1  PParamMin=[]  PParamMax=[]  IParamMin=[]  IParamMax=[]  DParamMin=[]  DParamMax=[]  NParamMin=[]  NParamMax=[]  KbParamMin=[]  KbParamMax=[]  KtParamMin=[]  KtParamMax=[]  POutMin=[]  POutMax=[]  IOutMin=[]  IOutMax=[]  DOutMin=[]  DOutMax=[]  NOutMin=[]  NOutMax=[]  KbOutMin=[]  KbOutMax=[]  KtOutMin=[]  KtOutMax=[]  IntegratorOutMin=[]  IntegratorOutMax=[]  FilterOutMin=[]  FilterOutMax=[]  SumOutMin=[]  SumOutMax=[]  SumI1OutMin=[]  SumI1OutMax=[]  SumI2OutMin=[]  SumI2OutMax=[]  SumI3OutMin=[]  SumI3OutMax=[]  SumDOutMin=[]  SumDOutMax=[]  SaturationOutMin=[]  SaturationOutMax=[]  IntegratorContinuousStateAttributes=''  IntegratorStateMustResolveToSignalObject=off  IntegratorRTWStateStorageClass=Auto  FilterContinuousStateAttributes=''  FilterStateMustResolveToSignalObject=off  FilterRTWStateStorageClass=Auto  DifferentiatorICPrevScaledInput=0  DifferentiatorOutMin=[]  DifferentiatorOutMax=[]  InitialConditionSetting=State (most efficient)
  PID Controller1 : simulink/Continuous/PID Controller  Controller=PID  TimeDomain=Continuous-time  SampleTime=-1  IntegratorMethod=Forward Euler  FilterMethod=Forward Euler  Form=Parallel  UseFilter=on  ControllerParametersSource=internal  P=0  I=-1  D=0  N=100  InitialConditionSource=internal  InitialConditionForIntegrator=0  InitialConditionForFilter=0  ExternalReset=none  LimitOutput=off  UpperSaturationLimit=inf  LowerSaturationLimit=-inf  LinearizeAsGain=on  AntiWindupMode=none  Kb=1  TrackingMode=off  Kt=1  PParamMin=[]  PParamMax=[]  IParamMin=[]  IParamMax=[]  DParamMin=[]  DParamMax=[]  NParamMin=[]  NParamMax=[]  KbParamMin=[]  KbParamMax=[]  KtParamMin=[]  KtParamMax=[]  POutMin=[]  POutMax=[]  IOutMin=[]  IOutMax=[]  DOutMin=[]  DOutMax=[]  NOutMin=[]  NOutMax=[]  KbOutMin=[]  KbOutMax=[]  KtOutMin=[]  KtOutMax=[]  IntegratorOutMin=[]  IntegratorOutMax=[]  FilterOutMin=[]  FilterOutMax=[]  SumOutMin=[]  SumOutMax=[]  SumI1OutMin=[]  SumI1OutMax=[]  SumI2OutMin=[]  SumI2OutMax=[]  SumI3OutMin=[]  SumI3OutMax=[]  SumDOutMin=[]  SumDOutMax=[]  SaturationOutMin=[]  SaturationOutMax=[]  IntegratorContinuousStateAttributes=''  IntegratorStateMustResolveToSignalObject=off  IntegratorRTWStateStorageClass=Auto  FilterContinuousStateAttributes=''  FilterStateMustResolveToSignalObject=off  FilterRTWStateStorageClass=Auto  DifferentiatorICPrevScaledInput=0  DifferentiatorOutMin=[]  DifferentiatorOutMax=[]  InitialConditionSetting=State (most efficient)
  Quat2Euler 1 : MATLAB Function  TreatAsAtomicUnit=on
  Quaternion Division : aerolibutil/Quaternion Division
      settings: SourceProductName=Aerospace Blockset  SourceProductBaseCode=AE
  Quaternion Normalize : sharedutil/Quaternion Normalize
  Scope : Scope
  Scope1 : Scope  Commented=on
  Scope2 : Scope  Commented=on
  Scope3 : Scope
  Sum : Sum  Commented=on  Inputs=|++
  Sum1 : Sum  Commented=on  Inputs=|+-
  Sum2 : Sum  Inputs=|+-
  Sum3 : Sum  Inputs=|++
  ATT_1 : Outport
  ATT_quat : Outport  Port=2
  wires:
  om_B_B_BE/1 -> Demux1/1, Matrix Multiply1/2, Matrix Multiply/2
  Integrator/1 -> Sum3/2, Sum2/2, Scope/1, ATT_1/1, Demux/1
  "Euler to Quat "/1(H) -> Matrix Multiply/1
  Theta_ini/1 -> Euler to Quat 3/1(att), Integrator/2, Integrator1/2  "Theta_ini"
  Matrix Multiply/1 -> Integrator/1
  Demux/3 -> Sum/2, Mux/2
  Demux/1 -> Mux1/1
  PID Controller/1 -> Sum1/2, Mux/1, Mux1/3
  Mux/1 -> Scope1/1
  Demux/2 -> Mux1/2
  Mux1/1 -> Scope2/1
  ROLL desire/1 -> Sum1/1
  Sum1/1 -> Sum/1
  Sum/1 -> PID Controller/1
  Sum2/1 -> PID Controller1/1
  ROLL desire1/1 -> Sum2/1
  PID Controller1/1 -> Sum3/1
  Sum3/1 -> "Euler to Quat "/1(att)
  Integrator1/1 -> Euler to Quat 1/1(att), Scope3/1
  Matrix Multiply1/1 -> Integrator1/1
  Euler to Quat 1/1(H) -> Matrix Multiply1/1
  Quaternion Normalize/1 -> Quat2Euler 1/1(Q), Quaternion Division/1
  Demux1/3 -> Mux2/4
  Integrator2/1 -> Quaternion Normalize/1
  Demux1/1 -> Mux2/2
  Quaternion Division/1 -> Gain/1
  Constant/1 -> Mux2/1
  Gain/1 -> Integrator2/1
  Mux2/1 -> Quaternion Division/2
  Demux1/2 -> Mux2/3
  Quat2Euler 1/1(theta) -> ATT_quat/1
  Euler to Quat 3/1(Q) -> Integrator2/2

== system FlightGear_BUS_aerosurface_trim/Subsystem/Subsystem ==
  In1 : Inport
  Demux : Demux  Outputs=3
  Gain : Gain  Gain=180/pi
  Mux : Mux  Inputs=2
  Terminator : Terminator
  Out1 : Outport
  wires:
  In1/1 -> Gain/1
  Demux/2 -> Mux/1
  Demux/3 -> Mux/2
  Mux/1 -> Out1/1
  Demux/1 -> Terminator/1
  Gain/1 -> Demux/1

== system FlightGear_BUS_aerosurface_trim/Subsystem/Trans Dyn1 ==
  Fext_B : Inport
  g_B : Inport  Port=2
  om_B_B_BE : Inport  Port=3
  m : Inport  Port=4
  V_initi : Inport  Port=5
  Add : Sum  Inputs=++-
  Cross Product : vrlib/Utilities/Cross Product
      settings: SourceProductBaseCode=VR
  Divide : Product  Inputs=*/
  Integrator : Integrator  InitialConditionSource=external
  Xdot_E_B_BE : Outport
  wires:
  Fext_B/1 -> Divide/1
  m/1 -> Divide/2
  Divide/1 -> Add/1
  g_B/1 -> Add/2
  om_B_B_BE/1 -> Cross Product/1
  Cross Product/1 -> Add/3
  Add/1 -> Integrator/1
  V_initi/1 -> Integrator/2
  Integrator/1 -> Cross Product/2, Xdot_E_B_BE/1

== system FlightGear_BUS_aerosurface_trim/Subsystem/atmosphere ==
  C_BN : Inport
  v_N_AE(wind NED) : Inport  Port=2
  Matrix Multiply : Product  Multiplication=Matrix(*)
  v_B_AE : Outport
  wires:
  v_N_AE(wind NED)/1 -> Matrix Multiply/2
  C_BN/1 -> Matrix Multiply/1
  Matrix Multiply/1 -> v_B_AE/1

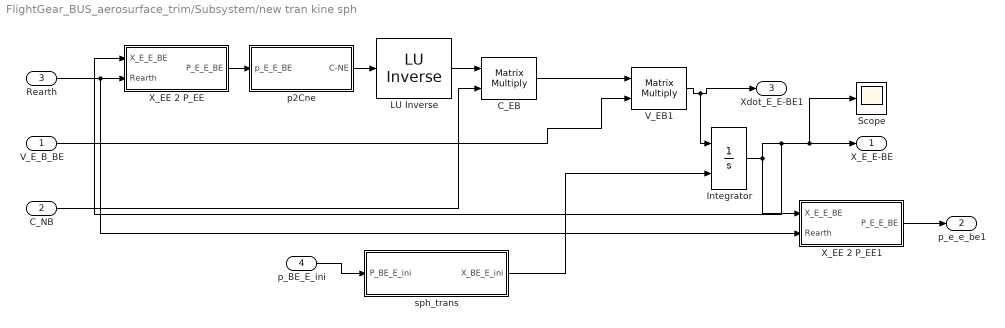
== system FlightGear_BUS_aerosurface_trim/Subsystem/new tran kine sph ==
  V_E_B_BE : Inport
  C_NB : Inport  Port=2
  Rearth : Inport  Port=3
  p_BE_E_ini : Inport  Port=4
  " LU Inverse" : dspinverses/ LU Inverse
      settings: SourceProductName=DSP System Toolbox
  C_EB : Product  Multiplication=Matrix(*)
  Integrator : Integrator  InitialConditionSource=external
  Scope : Scope
  V_EB1 : Product  Multiplication=Matrix(*)
  X_EE 2 P_EE : Subsystem
  X_EE 2 P_EE1 : Subsystem
  p2Cne : Subsystem
  sph_trans : MATLAB Function  TreatAsAtomicUnit=on
  X_E_E-BE : Outport
  p_e_e_be1 : Outport  Port=2
  Xdot_E_E-BE1 : Outport  Port=3
  wires:
  " LU Inverse"/1 -> C_EB/1
  Integrator/1 -> Scope/1, X_E_E-BE/1, X_EE 2 P_EE/1(X_E_E_BE), X_EE 2 P_EE1/1(X_E_E_BE)
  X_EE 2 P_EE1/1(P_E_E_BE) -> p_e_e_be1/1
  Rearth/1 -> X_EE 2 P_EE1/2(Rearth), X_EE 2 P_EE/2(Rearth)
  V_EB1/1 -> Xdot_E_E-BE1/1, Integrator/1
  C_EB/1 -> V_EB1/1
  p2Cne/1(C-NE) -> " LU Inverse"/1
  X_EE 2 P_EE/1(P_E_E_BE) -> p2Cne/1(p_E_E_BE)
  C_NB/1 -> C_EB/2
  V_E_B_BE/1 -> V_EB1/2
  p_BE_E_ini/1 -> sph_trans/1(P_BE_E_ini)
  sph_trans/1(X_BE_E_ini) -> Integrator/2

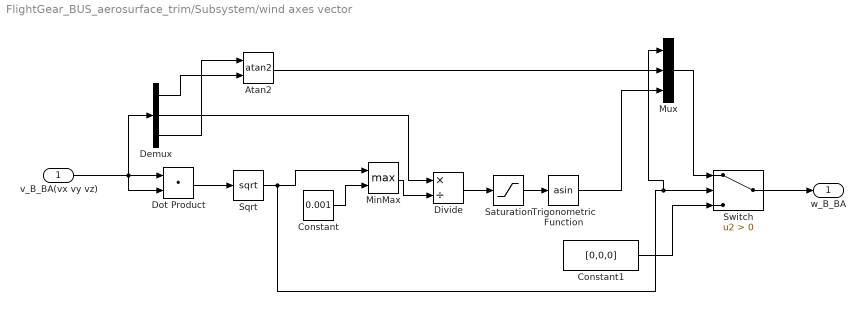
== system FlightGear_BUS_aerosurface_trim/Subsystem/wind axes vector ==
  v_B_BA(vx vy vz) : Inport
  Atan2 : Trigonometry  Operator=atan2
  Constant : Constant  Value=0.001
  Constant1 : Constant  Value=[0,0,0]
  Demux : Demux  Outputs=3
  Divide : Product  Inputs=*/
  Dot Product : DotProduct  InputSameDT=on  OutDataTypeStr=Inherit: Inherit via internal rule
  MinMax : MinMax  Function=max  Inputs=2
  Mux : Mux  Inputs=3
  Saturation : Saturate
  Sqrt : Sqrt  SaturateOnIntegerOverflow=on
  Switch : Switch  Criteria=u2 > Threshold
  Trigonometric Function : Trigonometry  Operator=asin  ApproximationMethod=CORDIC
  w_B_BA : Outport
  wires:
  v_B_BA(vx vy vz)/1 -> Demux/1, Dot Product/2, Dot Product/1
  Dot Product/1 -> Sqrt/1
  Sqrt/1 -> Mux/1, Switch/2, MinMax/1
  Constant/1 -> MinMax/2
  MinMax/1 -> Divide/2
  Demux/2 -> Divide/1
  Demux/3 -> Atan2/1
  Demux/1 -> Atan2/2
  Atan2/1 -> Mux/2
  Divide/1 -> Saturation/1
  Saturation/1 -> Trigonometric Function/1
  Trigonometric Function/1 -> Mux/3
  Constant1/1 -> Switch/3
  Mux/1 -> Switch/1
  Switch/1 -> w_B_BA/1

== system FlightGear_BUS_aerosurface_trim/new tran kine sph/X_EE 2 P_EE ==
  X_E_E_BE : Inport
  Rearth : Inport  Port=2
  Add : Sum  Inputs=+-
  Atan1 : Trigonometry  Operator=asin
  Atan2 : Trigonometry  Operator=atan2
  Demux : Demux  Outputs=3
  Divide : Product  Inputs=*/
  Dot Product1 : DotProduct  InputSameDT=on  OutDataTypeStr=Inherit: Inherit via internal rule
  Mux1 : Mux  Inputs=3
  Signed Sqrt1 : Sqrt  SaturateOnIntegerOverflow=on
  P_E_E_BE : Outport
  wires:
  X_E_E_BE/1 -> Dot Product1/2, Dot Product1/1, Demux/1
  Demux/1 -> Atan2/2
  Demux/2 -> Atan2/1
  Atan2/1 -> Mux1/2
  Dot Product1/1 -> Signed Sqrt1/1
  Signed Sqrt1/1 -> Add/1
  Rearth/1 -> Divide/2, Add/2
  Add/1 -> Mux1/3
  Mux1/1 -> P_E_E_BE/1
  Demux/3 -> Divide/1
  Divide/1 -> Atan1/1
  Atan1/1 -> Mux1/1

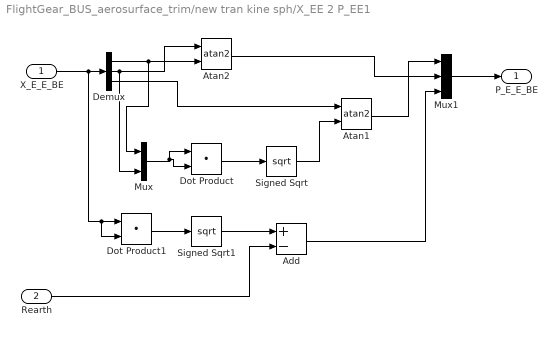
== system FlightGear_BUS_aerosurface_trim/new tran kine sph/X_EE 2 P_EE1 ==
  X_E_E_BE : Inport
  Rearth : Inport  Port=2
  Add : Sum  Inputs=+-
  Atan1 : Trigonometry  Operator=atan2
  Atan2 : Trigonometry  Operator=atan2
  Demux : Demux  Outputs=3
  Dot Product : DotProduct  InputSameDT=on  OutDataTypeStr=Inherit: Inherit via internal rule
  Dot Product1 : DotProduct  InputSameDT=on  OutDataTypeStr=Inherit: Inherit via internal rule
  Mux : Mux  Inputs=2
  Mux1 : Mux  Inputs=3
  Signed Sqrt : Sqrt  SaturateOnIntegerOverflow=on
  Signed Sqrt1 : Sqrt  SaturateOnIntegerOverflow=on
  P_E_E_BE : Outport
  wires:
  X_E_E_BE/1 -> Dot Product1/2, Dot Product1/1, Demux/1
  Demux/1 -> Mux/1, Atan2/2
  Demux/2 -> Atan2/1, Mux/2
  Mux/1 -> Dot Product/2, Dot Product/1
  Dot Product/1 -> Signed Sqrt/1
  Signed Sqrt/1 -> Atan1/2
  Demux/3 -> Atan1/1
  Atan2/1 -> Mux1/2
  Atan1/1 -> Mux1/1
  Dot Product1/1 -> Signed Sqrt1/1
  Signed Sqrt1/1 -> Add/1
  Rearth/1 -> Add/2
  Add/1 -> Mux1/3
  Mux1/1 -> P_E_E_BE/1

== system FlightGear_BUS_aerosurface_trim/new tran kine sph/p2Cne ==
  p_E_E_BE : Inport
  Constant : Constant  Value=[0 0 1; 0 1 0;-1 0 0]
  Demux : Demux  Outputs=3
  LAT DCM : MATLAB Function  TreatAsAtomicUnit=on
  LON DCM : MATLAB Function  TreatAsAtomicUnit=on
  Matrix Multiply : Product  Multiplication=Matrix(*)
  Matrix Multiply1 : Product  Multiplication=Matrix(*)
  Scope1 : Scope
  Terminator : Terminator
  C-NE : Outport
  wires:
  p_E_E_BE/1 -> Demux/1
  Demux/3 -> Terminator/1
  Demux/2 -> LON DCM/1(u)
  Demux/1 -> LAT DCM/1(u)
  LAT DCM/1(y) -> Matrix Multiply/1
  LON DCM/1(y) -> Matrix Multiply/2
  Matrix Multiply/1 -> Matrix Multiply1/1
  Constant/1 -> Matrix Multiply1/2
  Matrix Multiply1/1 -> Scope1/1, C-NE/1

== system FlightGear_BUS_aerosurface_trim/Subsystem/new tran kine sph/X_EE 2 P_EE ==
  X_E_E_BE : Inport
  Rearth : Inport  Port=2
  Add : Sum  Inputs=+-
  Atan1 : Trigonometry  Operator=asin
  Atan2 : Trigonometry  Operator=atan2
  Demux : Demux  Outputs=3
  Divide : Product  Inputs=*/
  Dot Product1 : DotProduct  InputSameDT=on  OutDataTypeStr=Inherit: Inherit via internal rule
  Mux1 : Mux  Inputs=3
  Signed Sqrt1 : Sqrt  SaturateOnIntegerOverflow=on
  P_E_E_BE : Outport
  wires:
  X_E_E_BE/1 -> Dot Product1/2, Dot Product1/1, Demux/1
  Demux/1 -> Atan2/2
  Demux/2 -> Atan2/1
  Atan2/1 -> Mux1/2
  Dot Product1/1 -> Signed Sqrt1/1
  Signed Sqrt1/1 -> Add/1
  Rearth/1 -> Divide/2, Add/2
  Add/1 -> Mux1/3
  Mux1/1 -> P_E_E_BE/1
  Demux/3 -> Divide/1
  Divide/1 -> Atan1/1
  Atan1/1 -> Mux1/1

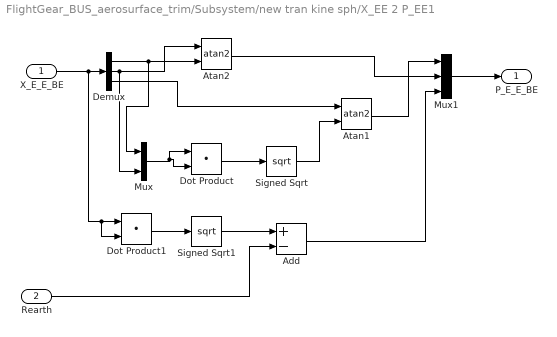
== system FlightGear_BUS_aerosurface_trim/Subsystem/new tran kine sph/X_EE 2 P_EE1 ==
  X_E_E_BE : Inport
  Rearth : Inport  Port=2
  Add : Sum  Inputs=+-
  Atan1 : Trigonometry  Operator=atan2
  Atan2 : Trigonometry  Operator=atan2
  Demux : Demux  Outputs=3
  Dot Product : DotProduct  InputSameDT=on  OutDataTypeStr=Inherit: Inherit via internal rule
  Dot Product1 : DotProduct  InputSameDT=on  OutDataTypeStr=Inherit: Inherit via internal rule
  Mux : Mux  Inputs=2
  Mux1 : Mux  Inputs=3
  Signed Sqrt : Sqrt  SaturateOnIntegerOverflow=on
  Signed Sqrt1 : Sqrt  SaturateOnIntegerOverflow=on
  P_E_E_BE : Outport
  wires:
  X_E_E_BE/1 -> Dot Product1/2, Dot Product1/1, Demux/1
  Demux/1 -> Mux/1, Atan2/2
  Demux/2 -> Atan2/1, Mux/2
  Mux/1 -> Dot Product/2, Dot Product/1
  Dot Product/1 -> Signed Sqrt/1
  Signed Sqrt/1 -> Atan1/2
  Demux/3 -> Atan1/1
  Atan2/1 -> Mux1/2
  Atan1/1 -> Mux1/1
  Dot Product1/1 -> Signed Sqrt1/1
  Signed Sqrt1/1 -> Add/1
  Rearth/1 -> Add/2
  Add/1 -> Mux1/3
  Mux1/1 -> P_E_E_BE/1

== system FlightGear_BUS_aerosurface_trim/Subsystem/new tran kine sph/p2Cne ==
  p_E_E_BE : Inport
  Constant : Constant  Value=[0 0 1; 0 1 0;-1 0 0]
  Demux : Demux  Outputs=3
  LAT DCM : MATLAB Function  TreatAsAtomicUnit=on
  LON DCM : MATLAB Function  TreatAsAtomicUnit=on
  Matrix Multiply : Product  Multiplication=Matrix(*)
  Matrix Multiply1 : Product  Multiplication=Matrix(*)
  Scope1 : Scope
  Terminator : Terminator
  C-NE : Outport
  wires:
  p_E_E_BE/1 -> Demux/1
  Demux/3 -> Terminator/1
  Demux/2 -> LON DCM/1(u)
  Demux/1 -> LAT DCM/1(u)
  LAT DCM/1(y) -> Matrix Multiply/1
  LON DCM/1(y) -> Matrix Multiply/2
  Matrix Multiply/1 -> Matrix Multiply1/1
  Constant/1 -> Matrix Multiply1/2
  Matrix Multiply1/1 -> Scope1/1, C-NE/1

== matlab function FlightGear_BUS_aerosurface_trim/new tran kine sph/p2Cne/LAT DCM ==
  data: u input; y output
function y = fcn(u)
y = [cos(u) 0 sin(u); 0 1 0; -sin(u) 0 cos(u)];

== matlab function FlightGear_BUS_aerosurface_trim/Rot kine/Euler to Quat 1 ==
  data: att input; H output
function H = fcn(att)
%#codegen
phi=att(1);
theta=att(2);
%psi=theta(3); %not needed for Euler Rotational Kinematics Matrix
H=[1,tan(theta)*sin(phi),tan(theta)*cos(phi); 0,cos(phi),-sin(phi);0,sin(phi)/cos(theta),cos(phi)/cos(theta)];

== matlab function FlightGear_BUS_aerosurface_trim/new tran kine sph/p2Cne/LON DCM ==
  data: u input; y output
function y = fcn(u)

y = [1, 0, 0;0, cos(u), sin(u);0, -sin(u), cos(u)];

== matlab function FlightGear_BUS_aerosurface_trim/AeroSurface controller/MATLAB Function ==
  data: V_B_BA input; V_inf input; F_b output; alp input; bet input; M_b output; CLa parameter; i_s2345 parameter; CL0_2345 parameter; a0_s2345 parameter; e_s2345 parameter; CDa_s2345 parameter; CD0_s2345 parameter; CM0_s2345 parameter; A_2345 parameter; xyz_s parameter; r parameter; CMa_s2345 parameter; c_2345 parameter; aileron_r input; aileron_l input; elevator input; rudder input
function [F_b, M_b] = fcn(V_B_BA,V_inf, alp,bet, CLa, i_s2345, CL0_2345, a0_s2345, e_s2345, CDa_s2345, CD0_s2345, CM0_s2345, A_2345, xyz_s, r, CMa_s2345, c_2345, aileron_r, aileron_l, elevator, rudder)
%% Properties
% CLa=2*pi*(r./(2+r)); 
% % V_B_BA=[ 1 1 1];V_inf=norm(V_B_BA); 
V_B_BA_0=[ V_B_BA(1); V_B_BA(2); V_B_BA(3)];
n1=[0,0,-1]; n2=[0,1,0]; n3=[0,0,-1]; n4=[0,0,-1]; 


a_ss1=i_s2345(1)-asin(complex(V_B_BA_0*n1)/V_inf);
a_ss2=i_s2345(2)-asin(complex(V_B_BA_0*n2)/V_inf);
a_ss3=i_s2345(3)-asin(complex(V_B_BA_0*n3)/V_inf);
a_ss4=i_s2345(4)-asin(complex(V_B_BA_0*n4)/V_inf);

a1=a_ss1-a0_s2345(1);
a2=a_ss2-a0_s2345(2);
a3=a_ss3-a0_s2345(3);
a4=a_ss4-a0_s2345(4);
%% for lift
CL1=CL0_2345(1)+CLa(1).*a_ss1+3*elevator*0.5;   %(0.075*0.35*0.2)/0.075*0.35; full span control surface
CL2=CL0_2345(2)+CLa(2).*a_ss2+3*rudder*0.5;   %(0.08*0.08*0.2)/(0.08*0.08); %Apply to fulsage(x*z) 
CL3=CL0_2345(3)+CLa(3).*a_ss3+3*aileron_r*0.5; %(0.02*0.96)/(0.1*0.96); 
CL4=CL0_2345(4)+CLa(4).*a_ss4+3*aileron_l*0.5;  %(0.02*0.96)/(0.1*0.96); %servo/wing

L1= CL1.*A_2345(1)*(0.5*(V_inf^2));
L2= CL2.*A_2345(2)*(0.5*(V_inf^2));
L3= CL3.*A_2345(3)*(0.5*(V_inf^2));
L4= CL4.*A_2345(4)*(0.5*(V_inf^2));


%% For Drag
cdl1=CL1.^2./(pi*(e_s2345(1).*r(1))); 
cdl2=CL2.^2./(pi*(e_s2345(2).*r(2))); 
cdl3=CL3.^2./(pi*(e_s2345(3).*r(3))); 
cdl4=CL4.^2./(pi*(e_s2345(4).*r(4)));

CD1=CD0_s2345(1)+CDa_s2345(1).*(a1.*a1)+cdl1;
CD2=CD0_s2345(2)+CDa_s2345(2).*(a2.*a2)+cdl2;
CD3=CD0_s2345(3)+CDa_s2345(3).*(a3.*a3)+cdl3;
CD4=CD0_s2345(4)+CDa_s2345(4).*(a4.*a4)+cdl4;

D1=CD1.*A_2345(1)*(0.5*V_inf.^2);
D2=CD2.*A_2345(2)*(0.5*V_inf.^2);
D3=CD3.*A_2345(3)*(0.5*V_inf.^2);
D4=CD4.*A_2345(4)*(0.5*V_inf.^2);
%% For moment
CM1=CM0_s2345(1)+CMa_s2345(1).*a_ss1;
CM2=CM0_s2345(2)+CMa_s2345(2).*a_ss2;
CM3=CM0_s2345(3)+CMa_s2345(3).*a_ss3;
CM4=CM0_s2345(4)+CMa_s2345(4).*a_ss4;
M1=CM1.*A_2345(1).*c_2345(1)*(0.5*V_inf.^2);
M2=CM2.*A_2345(2).*c_2345(2)*(0.5*V_inf.^2);
M3=CM3.*A_2345(3).*c_2345(3)*(0.5*V_inf.^2);
M4=CM4.*A_2345(4).*c_2345(4)*(0.5*V_inf.^2);

%% for fulsage
CD_f=0.5; %%% from 0.5 to 1
D_fulsage=CD_f.*0.001*(0.5*V_inf.^2);
F_fulsage=-[D_fulsage;0;0];

%% For F_b inner
n11=[0;0;-1]; n22=[0;1;0]; n33=[0;0;-1]; n44=[0;0;-1]; 
F_surf1=L1*n11-[norm(D1);0;0];
F_surf2=L2*n22-[norm(D2);0;0];
F_surf3=L3*n33-[norm(D3);0;0];
F_surf4=L4*n44-[norm(D4);0;0];

Csb=[cos(alp), 0, sin(alp); 0, 1,0; -1*sin(alp) 0 cos(alp)];
Cws=[cos(bet),sin(bet),0 ; -1*sin(bet),cos(bet),0;0, 0 ,1];
Cwb=Cws*Csb;
Cbw=inv(Cwb);


F_b1=Cbw*F_surf1;F_b2=Cbw*F_surf2;F_b3=Cbw*F_surf3;F_b4=Cbw*F_surf4;F_b5=Cbw*F_fulsage;
% F_surf=F_surf1+F_surf2+F_surf3+F_surf4+F_fulsage;

F_b=F_b1+F_b2+F_b3+F_b4+F_b5;

% c=cross(xyz_s(i,:),F_b(:,1));
C=[0,0,0;0,0,-1;0, 1,0];
% M_s2345=zeros(3,4);
T1=transpose(cross(xyz_s(1,:),F_b1));
T2=transpose(cross(xyz_s(2,:),F_b2));
T3=transpose(cross(xyz_s(3,:),F_b3));
T4=transpose(cross(xyz_s(4,:),F_b4));
M_b1=M1*C*n11+T1;
M_b2=M2*C*n22+T2;
M_b3=M3*C*n33+T3;
M_b4=M4*C*n44+T4;
M_b=M_b1+M_b2+M_b3+M_b4;
end

== matlab function FlightGear_BUS_aerosurface_trim/Subsystem/AeroSurface controller/MATLAB Function ==
  data: V_B_BA input; V_inf input; F_b output; alp input; bet input; M_b output; CLa parameter; i_s2345 parameter; CL0_2345 parameter; a0_s2345 parameter; e_s2345 parameter; CDa_s2345 parameter; CD0_s2345 parameter; CM0_s2345 parameter; A_2345 parameter; xyz_s parameter; r parameter; CMa_s2345 parameter; c_2345 parameter; aileron_r input; aileron_l input; elevator input; rudder input
function [F_b, M_b] = fcn(V_B_BA,V_inf, alp,bet, CLa, i_s2345, CL0_2345, a0_s2345, e_s2345, CDa_s2345, CD0_s2345, CM0_s2345, A_2345, xyz_s, r, CMa_s2345, c_2345, aileron_r, aileron_l, elevator, rudder)
%% Properties
% CLa=2*pi*(r./(2+r)); 
% % V_B_BA=[ 1 1 1];V_inf=norm(V_B_BA); 
V_B_BA_0=[ V_B_BA(1); V_B_BA(2); V_B_BA(3)];
n1=[0,0,-1]; n2=[0,1,0]; n3=[0,0,-1]; n4=[0,0,-1]; 


a_ss1=i_s2345(1)-asin(complex(V_B_BA_0*n1)/V_inf);
a_ss2=i_s2345(2)-asin(complex(V_B_BA_0*n2)/V_inf);
a_ss3=i_s2345(3)-asin(complex(V_B_BA_0*n3)/V_inf);
a_ss4=i_s2345(4)-asin(complex(V_B_BA_0*n4)/V_inf);

a1=a_ss1-a0_s2345(1);
a2=a_ss2-a0_s2345(2);
a3=a_ss3-a0_s2345(3);
a4=a_ss4-a0_s2345(4);
%% for lift
CL1=CL0_2345(1)+CLa(1).*a_ss1+3*elevator*0.5;   %(0.075*0.35*0.2)/0.075*0.35; full span control surface
CL2=CL0_2345(2)+CLa(2).*a_ss2+3*rudder*0.5;   %(0.08*0.08*0.2)/(0.08*0.08); %Apply to fulsage(x*z) 
CL3=CL0_2345(3)+CLa(3).*a_ss3+3*aileron_r*0.5; %(0.02*0.96)/(0.1*0.96); 
CL4=CL0_2345(4)+CLa(4).*a_ss4+3*aileron_l*0.5;  %(0.02*0.96)/(0.1*0.96); %servo/wing

L1= CL1.*A_2345(1)*(0.5*(V_inf^2));
L2= CL2.*A_2345(2)*(0.5*(V_inf^2));
L3= CL3.*A_2345(3)*(0.5*(V_inf^2));
L4= CL4.*A_2345(4)*(0.5*(V_inf^2));


%% For Drag
cdl1=CL1.^2./(pi*(e_s2345(1).*r(1))); 
cdl2=CL2.^2./(pi*(e_s2345(2).*r(2))); 
cdl3=CL3.^2./(pi*(e_s2345(3).*r(3))); 
cdl4=CL4.^2./(pi*(e_s2345(4).*r(4)));

CD1=CD0_s2345(1)+CDa_s2345(1).*(a1.*a1)+cdl1;
CD2=CD0_s2345(2)+CDa_s2345(2).*(a2.*a2)+cdl2;
CD3=CD0_s2345(3)+CDa_s2345(3).*(a3.*a3)+cdl3;
CD4=CD0_s2345(4)+CDa_s2345(4).*(a4.*a4)+cdl4;

D1=CD1.*A_2345(1)*(0.5*V_inf.^2);
D2=CD2.*A_2345(2)*(0.5*V_inf.^2);
D3=CD3.*A_2345(3)*(0.5*V_inf.^2);
D4=CD4.*A_2345(4)*(0.5*V_inf.^2);
%% For moment
CM1=CM0_s2345(1)+CMa_s2345(1).*a_ss1;
CM2=CM0_s2345(2)+CMa_s2345(2).*a_ss2;
CM3=CM0_s2345(3)+CMa_s2345(3).*a_ss3;
CM4=CM0_s2345(4)+CMa_s2345(4).*a_ss4;
M1=CM1.*A_2345(1).*c_2345(1)*(0.5*V_inf.^2);
M2=CM2.*A_2345(2).*c_2345(2)*(0.5*V_inf.^2);
M3=CM3.*A_2345(3).*c_2345(3)*(0.5*V_inf.^2);
M4=CM4.*A_2345(4).*c_2345(4)*(0.5*V_inf.^2);

%% for fulsage
CD_f=0.5; %%% from 0.5 to 1
D_fulsage=CD_f.*0.001*(0.5*V_inf.^2);
F_fulsage=-[D_fulsage;0;0];

%% For F_b inner
n11=[0;0;-1]; n22=[0;1;0]; n33=[0;0;-1]; n44=[0;0;-1]; 
F_surf1=L1*n11-[norm(D1);0;0];
F_surf2=L2*n22-[norm(D2);0;0];
F_surf3=L3*n33-[norm(D3);0;0];
F_surf4=L4*n44-[norm(D4);0;0];

Csb=[cos(alp), 0, sin(alp); 0, 1,0; -1*sin(alp) 0 cos(alp)];
Cws=[cos(bet),sin(bet),0 ; -1*sin(bet),cos(bet),0;0, 0 ,1];
Cwb=Cws*Csb;
Cbw=inv(Cwb);


F_b1=Cbw*F_surf1;F_b2=Cbw*F_surf2;F_b3=Cbw*F_surf3;F_b4=Cbw*F_surf4;F_b5=Cbw*F_fulsage;
% F_surf=F_surf1+F_surf2+F_surf3+F_surf4+F_fulsage;

F_b=F_b1+F_b2+F_b3+F_b4+F_b5;

% c=cross(xyz_s(i,:),F_b(:,1));
C=[0,0,0;0,0,-1;0, 1,0];
% M_s2345=zeros(3,4);
T1=transpose(cross(xyz_s(1,:),F_b1));
T2=transpose(cross(xyz_s(2,:),F_b2));
T3=transpose(cross(xyz_s(3,:),F_b3));
T4=transpose(cross(xyz_s(4,:),F_b4));
M_b1=M1*C*n11+T1;
M_b2=M2*C*n22+T2;
M_b3=M3*C*n33+T3;
M_b4=M4*C*n44+T4;
M_b=M_b1+M_b2+M_b3+M_b4;
end

== matlab function FlightGear_BUS_aerosurface_trim/Rot kine/Euler Angle  ==
  data: att input; H output
function H = fcn(att)
%#codegen
phi=att(1);
theta=att(2);
%psi=theta(3); %not needed for Euler Rotational Kinematics Matrix
H=[1,tan(theta)*sin(phi),tan(theta)*cos(phi); 0,cos(phi),-sin(phi);0,sin(phi)/cos(theta),cos(phi)/cos(theta)];

== matlab function FlightGear_BUS_aerosurface_trim/Subsystem/Rot kine/Euler to Quat  ==
  data: att input; H output
function H = fcn(att)
%#codegen
phi=att(1);
theta=att(2);
%psi=theta(3); %not needed for Euler Rotational Kinematics Matrix
H=[1,tan(theta)*sin(phi),tan(theta)*cos(phi); 0,cos(phi),-sin(phi);0,sin(phi)/cos(theta),cos(phi)/cos(theta)];
